simulink model "lab2_220726"  (R2016a)
settings: Solver=VariableStepAuto  StartTime=0.0  StopTime=10.0  RelTol=1e-3
settings Model: Creator=CSE  LastModifiedBy=CSE

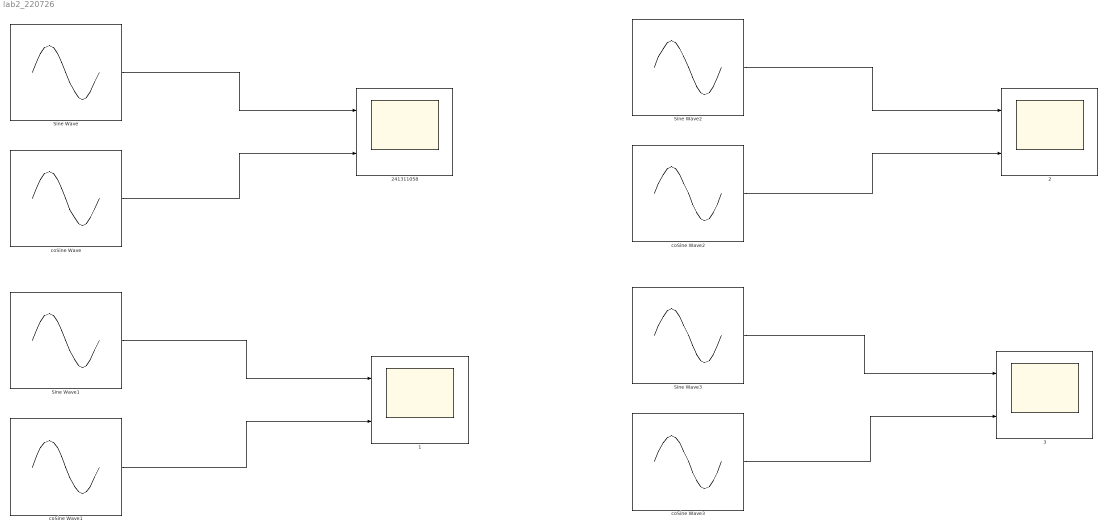
== system lab2_220726 ==
  {1..3,241311058} (4 alike) : Scope  NumInputPorts=2
  Sine Wave : Sin  SampleTime=0
  Sine Wave1 : Sin  Frequency=2  SampleTime=0
  Sine Wave2 : Sin  SampleTime=1e-3
  Sine Wave3 : Sin  Frequency=2  SampleTime=1e-3
  coSine Wave : Sin  Phase=pi/2  SampleTime=0
  coSine Wave1 : Sin  Phase=pi/2  SampleTime=0
  coSine Wave2 : Sin  Phase=pi/2  SampleTime=1e-3
  coSine Wave3 : Sin  Phase=pi/2  SampleTime=1e-3
  wires:
  Sine Wave/1 -> 241311058/1
  coSine Wave/1 -> 241311058/2
  Sine Wave1/1 -> 1/1
  coSine Wave1/1 -> 1/2
  Sine Wave2/1 -> 2/1
  coSine Wave2/1 -> 2/2
  Sine Wave3/1 -> 3/1
  coSine Wave3/1 -> 3/2
